simulink model "PickPlaceAdelanto"  (R2024a)
settings: Solver=VariableStepAuto  StartTime=0.0  StopTime=10  MaxStep=0.001  RelTol=1e-3
values from neighbouring files (symbols this model uses):
  AB = bandwidth(fdtLazoCerrado)    [PickandPlaceFrecuencia.m]
  Ka = 1    [PickandPlaceFrecuencia.m]
  T = Toscilante    [PickandPlaceFrecuencia.m]
settings Model: Creator=Ana  LastModifiedBy=Itsaso
settings ModelReferenceCC: EnableRefExpFcnMdlSchedulingChecks=on
settings RTWCC: GPUComputeCapability=3.5

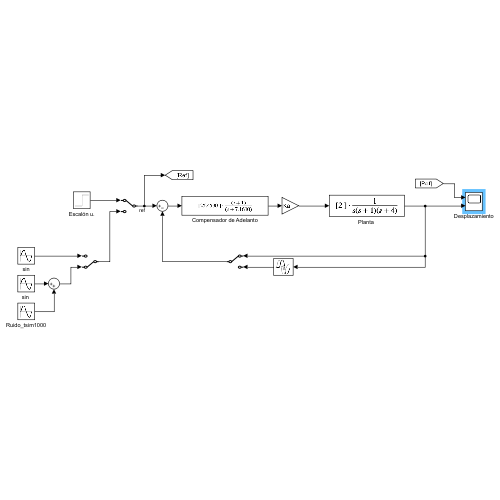
[thumbnail: Simulink's stored preview of the top-level diagram]
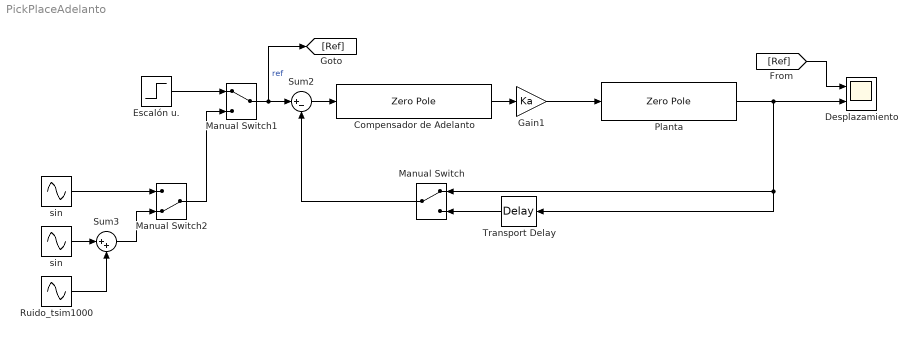
== system PickPlaceAdelanto ==
  Compensador de Adelanto : ZeroPole  Zeros=[-1]  Poles=[-7.1610]  Gain=[25.4530]
  Desplazamiento : Scope  NumInputPorts=2
  Escalón u. : Step  SampleTime=0
  Gain1 : Gain  Gain=Ka
  Manual Switch : ManualSwitch
  Manual Switch1 : ManualSwitch
  Manual Switch2 : ManualSwitch  CurrentSetting=0
  "Planta " : ZeroPole  Zeros=[]  Poles=[0 -1 -4]  Gain=[2]
  Ruido_tsim1000 : Sin  Amplitude=0.1  Frequency=10000  SampleTime=0
  Sum2 : Sum  Inputs=|+-  SaturateOnIntegerOverflow=on
  Sum3 : Sum  Inputs=|++
  Transport Delay : TransportDelay  DelayTime=T
  sin : Sin  Frequency=AB  SampleTime=0
  "sin " : Sin  Frequency=0.02  SampleTime=0
  wires:
  Manual Switch1/1 -> [Ref], Sum2/1  "ref"
  Ruido_tsim1000/1 -> Sum3/2
  Sum3/1 -> Manual Switch2/2
  "sin "/1 -> Sum3/1
  [Ref] -> Desplazamiento/1
  Manual Switch2/1 -> Manual Switch1/2
  sin/1 -> Manual Switch2/1
  Transport Delay/1 -> Manual Switch/2
  Manual Switch/1 -> Sum2/2
  Compensador de Adelanto/1 -> Gain1/1
  "Planta "/1 -> Manual Switch/1, Transport Delay/1, Desplazamiento/2
  Escalón u./1 -> Manual Switch1/1
  Sum2/1 -> Compensador de Adelanto/1
  Gain1/1 -> "Planta "/1
